simulink model "Starting_Position"  (R2015a)
settings: Solver=ode45  StartTime=0.0  StopTime=inf  FixedStep=0.002  RelTol=1e-3
values from neighbouring files (symbols this model uses):
  Ts = 0.06    [Parameters.m]
undefined symbols (not defined in the file or in its folder): DiscIntNeverNeededParam
libraries: arduino_io_lib x29, simulink x4
settings Model: CovMetricSettings=dwe  CovHtmlReporting=off  covSaveCumulativeToWorkspaceVar=off  CovSaveSingleToWorkspaceVar=off  CovExternalEMLEnable=on  ExtModeTrigDuration=10000  Creator=Antonio  LastModifiedBy=Antonio
settings SolverCC: PositivePriorityOrder=on
settings DataIOCC: LimitDataPoints=off  SaveFormat=Dataset
settings DebuggingCC: SFUnexpectedBacktrackingDiag=error  SFNoUnconditionalDefaultTransitionDiag=error
settings HardwareCC: ProdBitPerPointer=64  ProdLargestAtomicFloat=Float  ProdIntDivRoundTo=Zero  ProdEndianess=LittleEndian  ProdHWDeviceType=Specified
settings ModelReferenceCC: PropagateSignalLabelsOutOfModel=on
settings RTWCC: SystemTargetFile=quarc_win64.tlc  TemplateMakefile=quarc_default_tmf  Description=QUARC Win64 Target
settings STFCustomTargetCC: TargetLibSuffix=.lib  TargetPreCompLibLocation=C:\PROGRA~3\QUARC\lib\2017a\win64\release  TargetLangStandard=C99 (ISO)  GenerateSampleERTMain=off  ConcurrentExecutionCompliant=on  ERTCustomFileBanners=off  SupportNonInlinedSFcns=on  SupportVariableSizeSignals=off  MATLABClassNameForMDSCustomization=Simulink.SoftwareTarget.GRTCustomization  GRTInterface=on  SystemTargetFile=quarc_win64.tlc
settings GRTTargetCC: TargetPreCompLibLocation=C:\PROGRA~3\QUARC\lib\2017a\win64\release  TargetLangStandard=C99 (ISO)  ParMdlRefBuildCompliant=off  CompOptLevelCompliant=off  GeneratePreprocessorConditionals=Use local settings  CombineOutputUpdateFcns=off  MatFileLogging=off  CPPClassGenCompliant=off  GRTInterface=on  ExtMode=on  ExtModeMexFile=quarc_comm

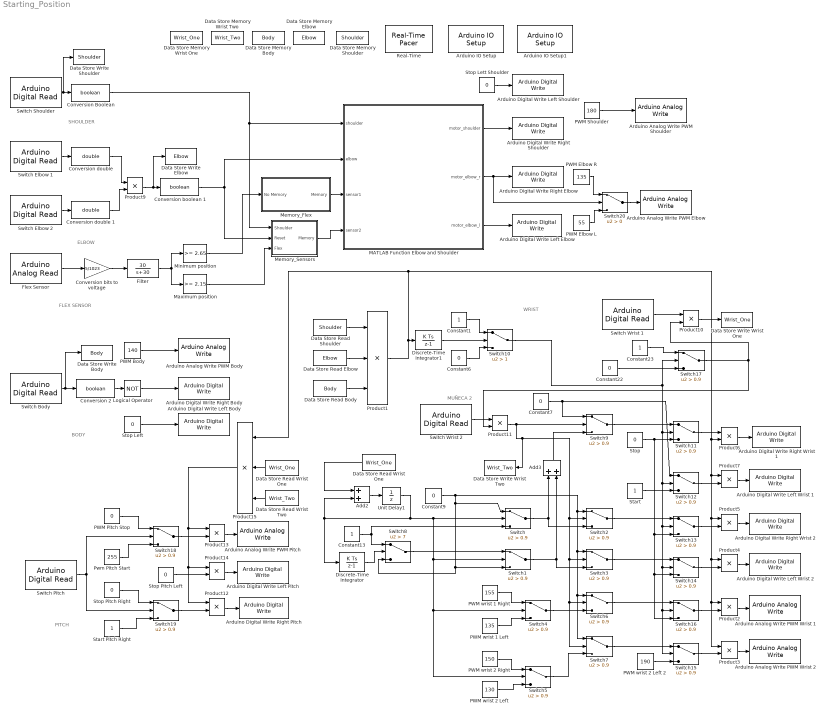
== system Starting_Position ==
  note: WRIST
  note: PITCH
  note: BODY
  note: SHOULDER
  note: MUÑECA 2
  note: FLEX SENSOR
  note: ELBOW
  Add2 : Sum
  Add3 : Sum
  Arduino Analog Write PWM Body : arduino_io_lib/Arduino Analog Write  arduinoVar=Temporary arduino variable: Arduino1  arduinoPin=9  T=Ts
  Arduino Analog Write PWM Elbow : arduino_io_lib/Arduino Analog Write  arduinoVar=Temporary arduino variable: Arduino1  arduinoPin=11  T=Ts
  Arduino Analog Write PWM Pitch : arduino_io_lib/Arduino Analog Write  arduinoVar=Temporary arduino variable: Arduino2  arduinoPin=9  T=Ts
  Arduino Analog Write PWM Shoulder : arduino_io_lib/Arduino Analog Write  arduinoVar=Temporary arduino variable: Arduino1  arduinoPin=10  T=Ts
  Arduino Analog Write PWM Wrist 1 : arduino_io_lib/Arduino Analog Write  arduinoVar=Temporary arduino variable: Arduino2  arduinoPin=11  T=Ts
  Arduino Analog Write PWM Wrist 2 : arduino_io_lib/Arduino Analog Write  arduinoVar=Temporary arduino variable: Arduino2  arduinoPin=10  T=Ts
  Arduino Digital Write Left Wrist 2 : arduino_io_lib/Arduino Digital Write  arduinoVar=Temporary arduino variable: Arduino2  arduinoPin=13  T=Ts
  Arduino Digital Write Right Wrist 1 : arduino_io_lib/Arduino Digital Write  arduinoVar=Temporary arduino variable: Arduino2  arduinoPin=5  T=Ts
  Arduino Digital Write Left Body : arduino_io_lib/Arduino Digital Write  arduinoVar=Temporary arduino variable: Arduino1  arduinoPin=7  T=Ts
  Arduino Digital Write Left Elbow : arduino_io_lib/Arduino Digital Write  arduinoVar=Temporary arduino variable: Arduino1  arduinoPin=12  T=Ts
  Arduino Digital Write Left Pitch : arduino_io_lib/Arduino Digital Write  arduinoVar=Temporary arduino variable: Arduino2  arduinoPin=6  T=Ts
  Arduino Digital Write Left Shoulder : arduino_io_lib/Arduino Digital Write  arduinoVar=Temporary arduino variable: Arduino1  arduinoPin=5  T=Ts
  Arduino Digital Write Left Wrist 1 : arduino_io_lib/Arduino Digital Write  arduinoVar=Temporary arduino variable: Arduino2  arduinoPin=4  T=Ts
  Arduino Digital Write Right Body : arduino_io_lib/Arduino Digital Write  arduinoVar=Temporary arduino variable: Arduino1  arduinoPin=6  T=Ts
  Arduino Digital Write Right Elbow : arduino_io_lib/Arduino Digital Write  arduinoVar=Temporary arduino variable: Arduino1  arduinoPin=13  T=Ts
  Arduino Digital Write Right Pitch : arduino_io_lib/Arduino Digital Write  arduinoVar=Temporary arduino variable: Arduino2  arduinoPin=7  T=Ts
  Arduino Digital Write Right Shoulder : arduino_io_lib/Arduino Digital Write  arduinoVar=Temporary arduino variable: Arduino1  arduinoPin=4  T=Ts
  Arduino Digital Write Right Wrist 2 : arduino_io_lib/Arduino Digital Write  arduinoVar=Temporary arduino variable: Arduino2  arduinoPin=12  T=Ts
  "Arduino IO Setup " : arduino_io_lib/Arduino IO Setup  Priority=3  arduinoVar=Temporary arduino variable: Arduino1  workspaceVarName=a  comPort=COM9
  Arduino IO Setup1 : arduino_io_lib/Arduino IO Setup  Priority=3  arduinoVar=Temporary arduino variable: Arduino2  workspaceVarName=a  comPort=COM3
  Constant1 : Constant
  Constant13 : Constant
  Constant{6..7,9,22} (4 alike) : Constant  Value=0
  Constant23 : Constant
  "Conversion 2 " : DataTypeConversion  OutDataTypeStr=boolean
  Conversion Boolean : DataTypeConversion  OutDataTypeStr=boolean
  Conversion bits to voltage : Gain  Gain=5/1023
  Conversion boolean 1 : DataTypeConversion  OutDataTypeStr=boolean
  Conversion double : DataTypeConversion  OutDataTypeStr=double
  "Conversion double 1 " : DataTypeConversion  OutDataTypeStr=double
  Data Store Memory Body : DataStoreMemory  DataStoreName=Body  ReadBeforeWriteMsg=warning  WriteAfterWriteMsg=warning  WriteAfterReadMsg=warning  ShowAdditionalParam=off
  Data Store Memory Elbow : DataStoreMemory  DataStoreName=Elbow  ReadBeforeWriteMsg=warning  WriteAfterWriteMsg=warning  WriteAfterReadMsg=warning  ShowAdditionalParam=off
  Data Store Memory Shoulder : DataStoreMemory  DataStoreName=Shoulder  ReadBeforeWriteMsg=warning  WriteAfterWriteMsg=warning  WriteAfterReadMsg=warning  ShowAdditionalParam=off
  Data Store Memory Wrist One : DataStoreMemory  DataStoreName=Wrist_One  ReadBeforeWriteMsg=warning  WriteAfterWriteMsg=warning  WriteAfterReadMsg=warning  ShowAdditionalParam=off
  Data Store Memory Wrist Two : DataStoreMemory  DataStoreName=Wrist_Two  ReadBeforeWriteMsg=warning  WriteAfterWriteMsg=warning  WriteAfterReadMsg=warning  ShowAdditionalParam=off
  Data Store Read Body : DataStoreRead  DataStoreName=Body
  Data Store Read Elbow : DataStoreRead  DataStoreName=Elbow
  Data Store Read Shoulder : DataStoreRead  DataStoreName=Shoulder
  Data Store Read Wrist One : DataStoreRead  DataStoreName=Wrist_One
  "Data Store Read Wrist One " : DataStoreRead  DataStoreName=Wrist_One
  Data Store Read Wrist Two : DataStoreRead  DataStoreName=Wrist_Two
  Data Store Write Body : DataStoreWrite  DataStoreName=Body
  Data Store Write Elbow : DataStoreWrite  DataStoreName=Elbow
  Data Store Write Shoulder : DataStoreWrite  DataStoreName=Shoulder
  Data Store Write Wrist One : DataStoreWrite  DataStoreName=Wrist_One
  "Data Store Write Wrist Two " : DataStoreWrite  DataStoreName=Wrist_Two
  Discrete-Time Integrator : DiscreteIntegrator  InitialConditionSetting=State (most efficient)  SampleTime=Ts  LimitOutput=on  UpperSaturationLimit=15  ICPrevOutput=DiscIntNeverNeededParam  ICPrevScaledInput=DiscIntNeverNeededParam
  Discrete-Time Integrator1 : DiscreteIntegrator  InitialConditionSetting=State (most efficient)  SampleTime=Ts  LimitOutput=on  UpperSaturationLimit=15  ICPrevOutput=DiscIntNeverNeededParam  ICPrevScaledInput=DiscIntNeverNeededParam
  "Filter " : TransferFcn  Numerator=[30]  Denominator=[1 30]
  "Flex Sensor " : arduino_io_lib/Arduino Analog Read  arduinoVar=Temporary arduino variable: Arduino2  arduinoPin=1  T=Ts
  Logical Operator : Logic  Operator=NOT  AllPortsSameDT=off  OutDataTypeStr=boolean
  MATLAB Function Elbow and Shoulder : MATLAB Function  TreatAsAtomicUnit=on
      settings: PermitHierarchicalResolution=ParametersOnly
  Maximum position : simulink/Logic and Bit Operations/Compare To Constant  relop=>=  const=2.15  OutDataTypeStr=boolean
  "Memory_Flex " : Subsystem
  Memory_Sensors : Subsystem
  Minimum position : simulink/Logic and Bit Operations/Compare To Constant  relop=>=  const=2.65  OutDataTypeStr=boolean
  PWM Body : Constant  Value=140
  PWM Elbow L : Constant  Value=55
  PWM Elbow R : Constant  Value=135
  PWM Pitch Stop : Constant  Value=0
  PWM Shoulder : Constant  Value=180
  PWM wrist 1 Left : Constant  Value=135
  PWM wrist 1 Right : Constant  Value=155
  PWM wrist 2 Left : Constant  Value=130
  PWM wrist 2 Left 2 : Constant  Value=190
  PWM wrist 2 Right : Constant  Value=150
  Product1 : Product  Inputs=3
  Product{2..7,9..14} (12 alike) : Product
  Product15 : Product  Inputs=3
  Pwm Pitch Start : Constant  Value=255
  "Real-Time " : arduino_io_lib/Real-Time Pacer  simTimePerRealTime=1
  Start : Constant
  Start Pitch Right : Constant
  Stop : Constant  Value=0
  Stop Left : Constant  Value=0
  Stop Lett Shoulder : Constant  Value=0
  "Stop Pitch Left " : Constant  Value=0
  Stop Pitch Right : Constant  Value=0
  Switch{,1..7,9,11..19} (18 alike) : Switch  Criteria=u2 > Threshold  Threshold=0.9
  Switch Body : arduino_io_lib/Arduino Digital Read  arduinoVar=Temporary arduino variable: Arduino2  arduinoPin=28  T=Ts
  Switch Elbow 1 : arduino_io_lib/Arduino Digital Read  arduinoVar=Temporary arduino variable: Arduino2  arduinoPin=22  T=Ts
  Switch Elbow 2 : arduino_io_lib/Arduino Digital Read  arduinoVar=Temporary arduino variable: Arduino2  arduinoPin=24  T=Ts
  "Switch Pitch " : arduino_io_lib/Arduino Digital Read  arduinoVar=Temporary arduino variable: Arduino2  arduinoPin=34  T=Ts
  Switch Shoulder : arduino_io_lib/Arduino Digital Read  arduinoVar=Temporary arduino variable: Arduino2  arduinoPin=26  T=Ts
  "Switch Wrist 1 " : arduino_io_lib/Arduino Digital Read  arduinoVar=Temporary arduino variable: Arduino2  arduinoPin=32  T=Ts
  "Switch Wrist 2 " : arduino_io_lib/Arduino Digital Read  arduinoVar=Temporary arduino variable: Arduino2  arduinoPin=30  T=Ts
  Switch10 : Switch  Criteria=u2 > Threshold  Threshold=1
  Switch20 : Switch  Criteria=u2 > Threshold
  Switch8 : Switch  Criteria=u2 > Threshold  Threshold=7
  Unit Delay1 : UnitDelay  SampleTime=Ts
  wires:
  MATLAB Function Elbow and Shoulder/1(motor_shoulder) -> Arduino Digital Write Right Shoulder/1
  Conversion boolean 1/1 -> Memory_Sensors/2(Reset), MATLAB Function Elbow and Shoulder/2(elbow)
  Conversion Boolean/1 -> Memory_Sensors/1(Shoulder), MATLAB Function Elbow and Shoulder/1(shoulder)
  MATLAB Function Elbow and Shoulder/3(motor_elbow_l) -> Arduino Digital Write Left Elbow/1
  Minimum position/1 -> "Memory_Flex "/1(No Memory)
  "Flex Sensor "/1 -> Conversion bits to voltage/1
  PWM Shoulder/1 -> Arduino Analog Write PWM Shoulder/1
  Stop Lett Shoulder/1 -> Arduino Digital Write Left Shoulder/1
  Switch Shoulder/1 -> Data Store Write Shoulder/1, Conversion Boolean/1
  Conversion double/1 -> Product9/1
  "Conversion double 1 "/1 -> Product9/2
  Switch Elbow 1/1 -> Conversion double/1
  Switch Elbow 2/1 -> "Conversion double 1 "/1
  Switch8/1 -> Switch1/1
  "Switch Pitch "/1 -> Switch18/2, Switch19/2
  Product5/1 -> Arduino Digital Write Right Wrist 2/1
  Pwm Pitch Start/1 -> Switch18/3
  Switch18/1 -> Product13/2
  Switch1/1 -> Switch3/3, Add3/2
  Product14/1 -> Arduino Digital Write Left Pitch/1
  Start/1 -> Switch12/3
  Product15/1 -> Product12/1, Product14/1, Product13/1
  Add2/1 -> Unit Delay1/1
  Product12/1 -> Arduino Digital Write Right Pitch/1
  Start Pitch Right/1 -> Switch19/3
  "Stop Pitch Left "/1 -> Product14/2
  Product11/1 -> "Data Store Write Wrist Two "/1, Switch2/2, Switch7/2, Switch6/2, Switch3/2, Switch9/2
  Stop Pitch Right/1 -> Switch19/1
  PWM Pitch Stop/1 -> Switch18/1
  Switch11/1 -> Product6/1
  Switch4/1 -> Switch6/3
  Switch6/1 -> Switch16/1
  Add3/1 -> Switch9/3
  Product2/1 -> Arduino Analog Write PWM Wrist 1/1
  PWM wrist 1 Right/1 -> Switch4/1
  Constant7/1 -> Switch9/1, Switch12/1
  Constant13/1 -> Switch/3, Switch8/1
  Discrete-Time Integrator1/1 -> Switch10/2
  Unit Delay1/1 -> Add2/2, Discrete-Time Integrator/1, Switch5/2, Switch4/2, Switch1/2, Switch/2
  Constant6/1 -> Switch10/3
  Switch9/1 -> Switch11/1
  Switch19/1 -> Product12/2
  Switch3/1 -> Switch14/1
  PWM wrist 2 Left/1 -> Switch5/3
  Switch10/1 -> Switch17/2, Switch11/2, Switch13/2, Switch15/2, Switch16/2, Switch14/2, Switch12/2
  Constant9/1 -> Switch7/1, Switch6/1, Switch3/1, Switch2/1, Switch8/3, Switch1/3, Switch/1
  Switch5/1 -> Switch7/3
  Product7/1 -> Arduino Digital Write Left Wrist 1/1
  Discrete-Time Integrator/1 -> Switch8/2
  Product6/1 -> Arduino Digital Write Right Wrist 1/1
  Constant22/1 -> Switch17/3
  Switch/1 -> Switch2/3, Add3/1
  PWM wrist 2 Left 2/1 -> Switch15/3
  Stop/1 -> Switch11/3, Switch14/3, Switch16/3, Switch13/3
  PWM wrist 1 Left/1 -> Switch4/3
  Product3/1 -> Arduino Analog Write PWM Wrist 2/1
  Switch14/1 -> Product4/2
  Switch2/1 -> Switch13/1
  PWM wrist 2 Right/1 -> Switch5/1
  Switch12/1 -> Product7/2
  Product13/1 -> Arduino Analog Write PWM Pitch/1
  Product1/1 -> Product6/2, Product7/1, Product5/1, Product2/1, Product3/1, Product4/1, Product15/1, Discrete-Time Integrator1/1
  Switch7/1 -> Switch15/1
  Constant23/1 -> Switch17/1
  Switch15/1 -> Product3/2
  "Switch Wrist 2 "/1 -> Product11/1
  Switch13/1 -> Product5/2
  Constant1/1 -> Switch10/1
  Switch16/1 -> Product2/2
  Product4/1 -> Arduino Digital Write Left Wrist 2/1
  Product9/1 -> Data Store Write Elbow/1, Conversion boolean 1/1
  MATLAB Function Elbow and Shoulder/2(motor_elbow_r) -> Switch20/2, Arduino Digital Write Right Elbow/1
  Conversion bits to voltage/1 -> "Filter "/1
  Switch Body/1 -> Data Store Write Body/1, "Conversion 2 "/1
  Stop Left/1 -> Arduino Digital Write Left Body/1
  PWM Body/1 -> Arduino Analog Write PWM Body/1
  "Conversion 2 "/1 -> Logical Operator/1
  "Memory_Flex "/1("Memory ") -> MATLAB Function Elbow and Shoulder/3(sensor1)
  Memory_Sensors/1(Memory) -> MATLAB Function Elbow and Shoulder/4(sensor2)
  "Switch Wrist 1 "/1 -> Product10/1
  Switch17/1 -> Product10/2, Product11/2
  Logical Operator/1 -> Arduino Digital Write Right Body/1
  Switch20/1 -> Arduino Analog Write PWM Elbow/1
  PWM Elbow R/1 -> Switch20/1
  PWM Elbow L/1 -> Switch20/3
  "Filter "/1 -> Maximum position/1, Minimum position/1
  Maximum position/1 -> Memory_Sensors/3(Flex)
  Data Store Read Shoulder/1 -> Product1/1
  Data Store Read Elbow/1 -> Product1/2
  Data Store Read Body/1 -> Product1/3
  Product10/1 -> Data Store Write Wrist One/1
  Data Store Read Wrist One/1 -> Product15/2
  "Data Store Read Wrist One "/1 -> Add2/1
  Data Store Read Wrist Two/1 -> Product15/3

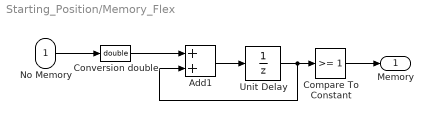
== system Starting_Position/Memory_Flex  ==
  No Memory : Inport
  Add1 : Sum
  Compare To Constant : simulink/Logic and Bit Operations/Compare To Constant  relop=>=  const=1  OutDataTypeStr=boolean
  Conversion double : DataTypeConversion  OutDataTypeStr=double
  Unit Delay : UnitDelay  SampleTime=Ts
  "Memory " : Outport
  wires:
  Compare To Constant/1 -> "Memory "/1
  Unit Delay/1 -> Add1/2, Compare To Constant/1
  Add1/1 -> Unit Delay/1
  Conversion double/1 -> Add1/1
  No Memory/1 -> Conversion double/1

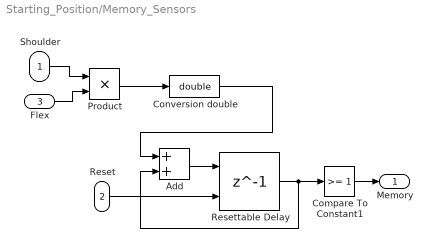
== system Starting_Position/Memory_Sensors ==
  Shoulder : Inport
  Reset : Inport  Port=2
  Flex : Inport  Port=3
  Add : Sum
  Compare To Constant1 : simulink/Logic and Bit Operations/Compare To Constant  relop=>=  const=1  OutDataTypeStr=boolean
  "Conversion double " : DataTypeConversion  OutDataTypeStr=double
  Product : Product
  Resettable Delay : Delay  DelayLength=1  ExternalReset=Rising  SampleTime=Ts
      settings: InputPortMap=u0,r5
  Memory : Outport
  wires:
  Add/1 -> Resettable Delay/1
  Resettable Delay/1 -> Add/2, Compare To Constant1/1
  Product/1 -> "Conversion double "/1
  Compare To Constant1/1 -> Memory/1
  "Conversion double "/1 -> Add/1
  Flex/1 -> Product/2
  Reset/1 -> Resettable Delay/2
  Shoulder/1 -> Product/1

== matlab function Starting_Position/MATLAB Function Elbow and Shoulder ==
  data: motor_shoulder output; shoulder input; motor_elbow_r output; elbow input; sensor1 input; motor_elbow_l output; sensor2 input
function [motor_shoulder,motor_elbow_r,motor_elbow_l]= fcn(shoulder,elbow,sensor1,sensor2)
%#codegen
motor_shoulder = 0;
motor_elbow_r = 0;
motor_elbow_l = 0;

%Conditional
if (shoulder==0 && sensor1==0)
  motor_shoulder = 0;
  motor_elbow_r = 1;
  motor_elbow_l = 0;
elseif (shoulder==0 && sensor1==1)
  motor_shoulder = 1;
  motor_elbow_r = 0;
  motor_elbow_l = 0;
elseif (shoulder==1 && elbow==0 && sensor2==0)
  motor_shoulder = 0;
  motor_elbow_r = 1;
  motor_elbow_l = 0;
elseif (shoulder==1 && elbow==0 && sensor2==1)
  motor_shoulder = 0;
  motor_elbow_r = 0;
  motor_elbow_l = 1;
elseif (shoulder==1 && elbow==1 && sensor2==0)
  motor_shoulder = 0;
  motor_elbow_r = 0;
  motor_elbow_l = 0;
end
